simulink library "csu_prb_orbit_perturbations_model_lib"  (R2014b)
settings: Solver=ode45  SolverMode=SingleTasking  StartTime=0.0  StopTime=10.0  RelTol=1e-3
values from neighbouring files (symbols this model uses):
  grv_mu_moon = gbl_param.moon_gravity_mu    [csu_grs_gravity_r_squared_init.m]
  ini_epoch_seconds = gbl_param.epoch_seconds    [csu_ini_initial_conditions_init.m]
undefined symbols (not defined in the file or in its folder): pos_s2m_mcmf, prb_gg_torque_on, prb_srp_force_on, r_moon, r_sun, spice_time_step_size, srp_K
libraries: util_common_lib x11, util_info_lib x7, util_quat_lib x4, csu_prb_orbit_perturbations_model_lib x2, csu_srp_solar_radiation_model_lib x1
settings Model: ExtModeAutoUpdateStatusClock=off  Creator=daniloviazzo  LastModifiedBy=mstewart

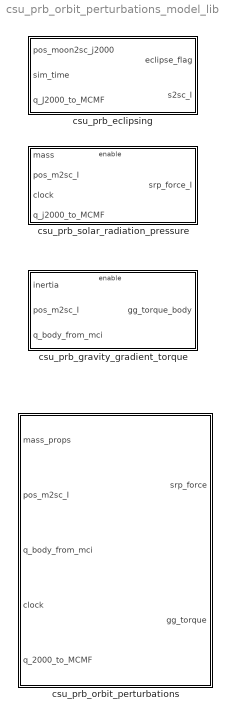
== system csu_prb_orbit_perturbations_model_lib ==
  csu_prb_eclipsing : Subsystem
  csu_prb_gravity_gradient_torque : Subsystem
  csu_prb_orbit_perturbations : Subsystem
  csu_prb_solar_radiation_pressure : Subsystem

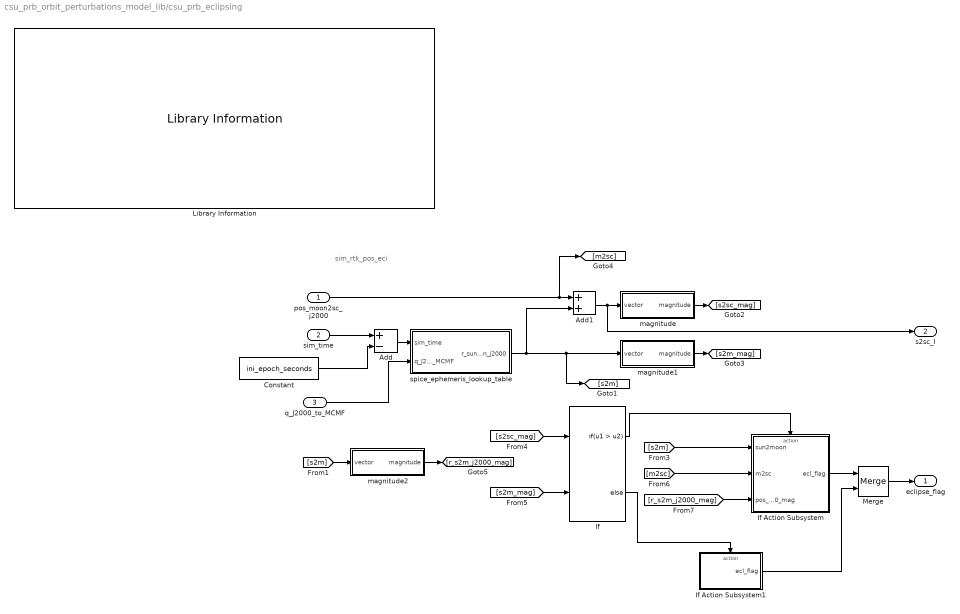
== system csu_prb_orbit_perturbations_model_lib/csu_prb_eclipsing ==
  note: sim_rtk_pos_eci
  pos_moon2sc_j2000 : Inport
  sim_time : Inport  Port=2
  q_J2000_to_MCMF : Inport  Port=3
  Add : Sum  Inputs=+-
  Add1 : Sum
  Constant : Constant  Value=ini_epoch_seconds
  If : If  NumInputs=2  IfExpression=u1 > u2
  If Action Subsystem : Subsystem  TreatAsAtomicUnit=on
  If Action Subsystem1 : Subsystem  TreatAsAtomicUnit=on
  Library Information : util_info_lib/Library Information  owner='NONE'
  Merge : Merge
  magnitude : Subsystem
  magnitude1 : Subsystem
  magnitude2 : Subsystem
  spice_ephemeris_lookup_table : Subsystem
  eclipse_flag : Outport
  s2sc_I : Outport  Port=2
  wires:
  [m2sc] -> If Action Subsystem/2(m2sc)
  [s2m_mag] -> If/2
  [s2sc_mag] -> If/1
  magnitude1/1(magnitude) -> [s2m_mag]
  magnitude/1(magnitude) -> [s2sc_mag]
  [s2m] -> If Action Subsystem/1(sun2moon)
  spice_ephemeris_lookup_table/1(r_sun2moon_j2000) -> magnitude1/1(vector), [s2m], Add1/2
  Add1/1 -> s2sc_I/1, magnitude/1(vector)
  Merge/1 -> eclipse_flag/1
  If Action Subsystem/1(ecl_flag) -> Merge/1
  If Action Subsystem1/1(ecl_flag) -> Merge/2
  If/2 -> If Action Subsystem1/Action
  If/1 -> If Action Subsystem/Action
  pos_moon2sc_j2000/1 -> [m2sc], Add1/1
  sim_time/1 -> Add/1
  Constant/1 -> Add/2
  Add/1 -> spice_ephemeris_lookup_table/1(sim_time)
  [r_s2m_j2000_mag] -> If Action Subsystem/3(pos_s2m_j2000_mag)
  q_J2000_to_MCMF/1 -> spice_ephemeris_lookup_table/2(q_J2000_to_MCMF)
  magnitude2/1(magnitude) -> [r_s2m_j2000_mag]
  [s2m] -> magnitude2/1(vector)

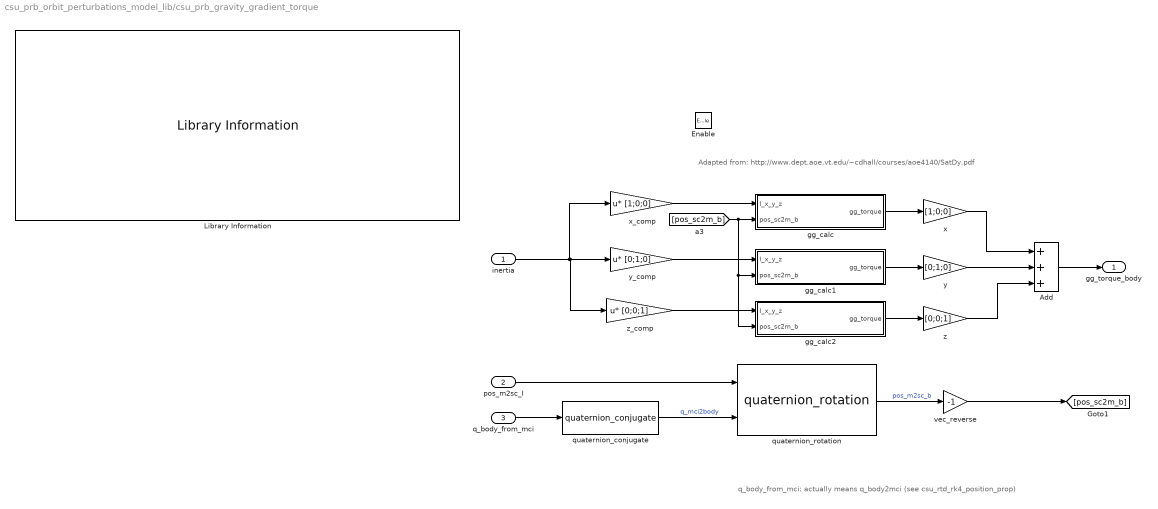
== system csu_prb_orbit_perturbations_model_lib/csu_prb_gravity_gradient_torque ==
  note: Adapted from: http://www.dept.aoe.vt.edu/~cdhall/courses/aoe4140/SatDy.pdf
  note: q_body_from_mci: actually means q_body2mci (see csu_rtd_rk4_position_prop)
  inertia : Inport
  pos_m2sc_I : Inport  Port=2
  q_body_from_mci : Inport  Port=3
  Enable : EnablePort
  Add : Sum  Inputs=+++
  Library Information : util_info_lib/Library Information  owner='NONE'
  gg_calc : Subsystem
  gg_calc1 : Subsystem
  gg_calc2 : Subsystem
  quaternion_conjugate : util_quat_lib/quaternion_conjugate  SystemSampleTime=-1
  quaternion_rotation : util_quat_lib/quaternion_rotation  SystemSampleTime=-1
  vec_reverse : Gain  Gain=-1
  x : Gain  Gain=[1;0;0]
  x_comp : Gain  Gain=[1;0;0]  Multiplication=Matrix(u*K)
  y : Gain  Gain=[0;1;0]
  y_comp : Gain  Gain=[0;1;0]  Multiplication=Matrix(u*K)
  z : Gain  Gain=[0;0;1]
  z_comp : Gain  Gain=[0;0;1]  Multiplication=Matrix(u*K)
  gg_torque_body : Outport
  wires:
  gg_calc2/1(gg_torque) -> z/1
  gg_calc1/1(gg_torque) -> y/1
  gg_calc/1(gg_torque) -> x/1
  [pos_sc2m_b] -> gg_calc/2(pos_sc2m_b), gg_calc1/2(pos_sc2m_b), gg_calc2/2(pos_sc2m_b)
  z_comp/1 -> gg_calc2/1(I_x_y_z)
  y_comp/1 -> gg_calc1/1(I_x_y_z)
  x_comp/1 -> gg_calc/1(I_x_y_z)
  Add/1 -> gg_torque_body/1
  inertia/1 -> y_comp/1, z_comp/1, x_comp/1
  vec_reverse/1 -> [pos_sc2m_b]
  quaternion_rotation/1 -> vec_reverse/1  "pos_m2sc_b"
  quaternion_conjugate/1 -> quaternion_rotation/2  "q_mci2body"
  q_body_from_mci/1 -> quaternion_conjugate/1
  pos_m2sc_I/1 -> quaternion_rotation/1
  x/1 -> Add/1
  y/1 -> Add/2
  z/1 -> Add/3

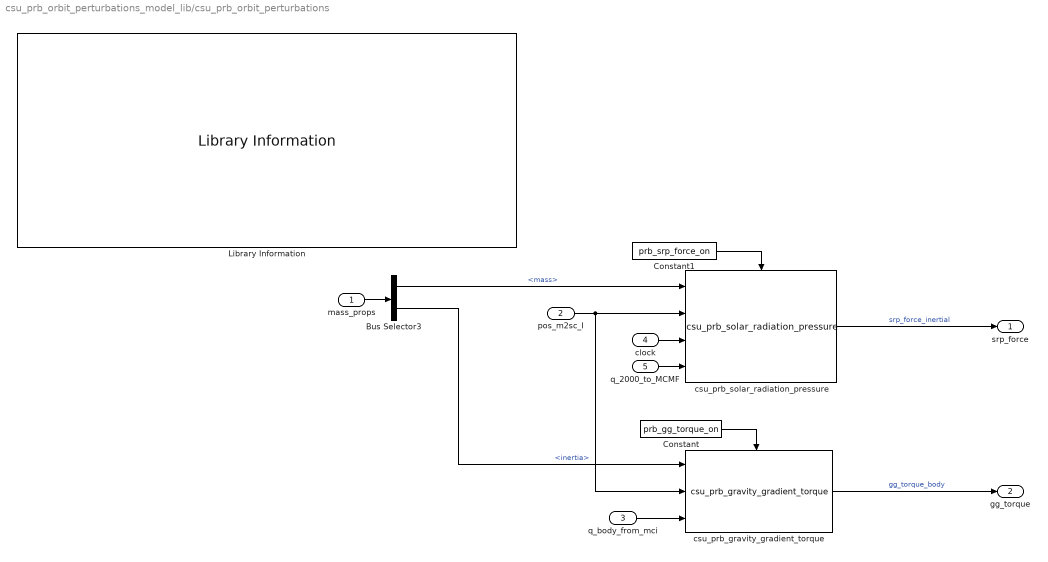
== system csu_prb_orbit_perturbations_model_lib/csu_prb_orbit_perturbations ==
  mass_props : Inport
  pos_m2sc_I : Inport  Port=2
  q_body_from_mci : Inport  Port=3
  clock : Inport  Port=4
  q_2000_to_MCMF : Inport  Port=5
  Bus Selector3 : BusSelector  OutputSignals=mass,inertia
  Constant : Constant  Value=prb_gg_torque_on
  Constant1 : Constant  Value=prb_srp_force_on
  Library Information : util_info_lib/Library Information  owner='NONE'
  csu_prb_gravity_gradient_torque : csu_prb_orbit_perturbations_model_lib/csu_prb_gravity_gradient_torque
  csu_prb_solar_radiation_pressure : csu_prb_orbit_perturbations_model_lib/csu_prb_solar_radiation_pressure
  srp_force : Outport
  gg_torque : Outport  Port=2
  wires:
  Bus Selector3/1 -> csu_prb_solar_radiation_pressure/1  "<mass>"
  mass_props/1 -> Bus Selector3/1
  q_2000_to_MCMF/1 -> csu_prb_solar_radiation_pressure/4
  clock/1 -> csu_prb_solar_radiation_pressure/3
  pos_m2sc_I/1 -> csu_prb_solar_radiation_pressure/2, csu_prb_gravity_gradient_torque/2
  q_body_from_mci/1 -> csu_prb_gravity_gradient_torque/3
  Constant/1 -> csu_prb_gravity_gradient_torque/Enable
  Constant1/1 -> csu_prb_solar_radiation_pressure/Enable
  Bus Selector3/2 -> csu_prb_gravity_gradient_torque/1  "<inertia>"
  csu_prb_solar_radiation_pressure/1 -> srp_force/1  "srp_force_inertial"
  csu_prb_gravity_gradient_torque/1 -> gg_torque/1  "gg_torque_body"

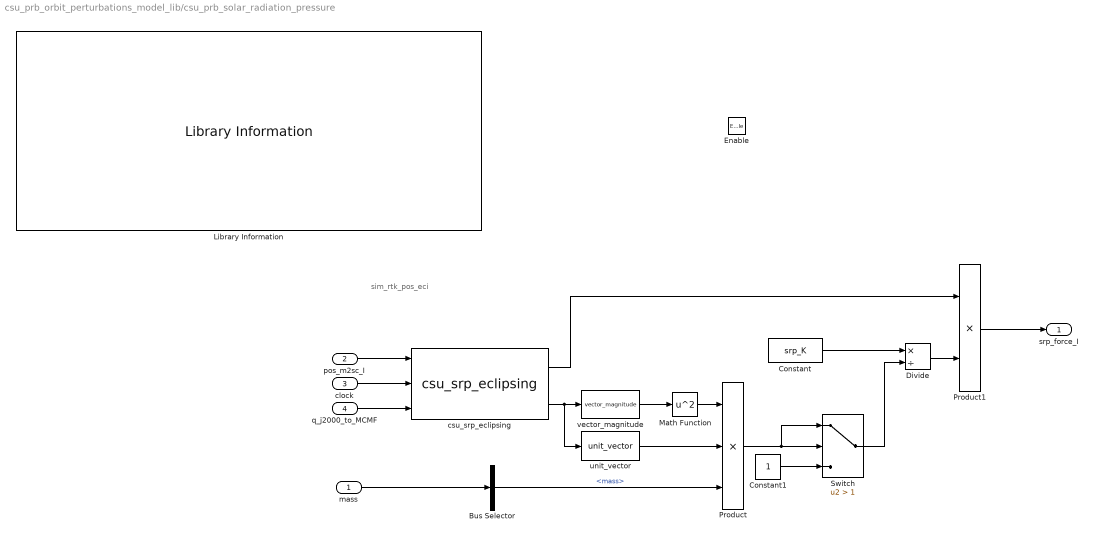
== system csu_prb_orbit_perturbations_model_lib/csu_prb_solar_radiation_pressure ==
  note: sim_rtk_pos_eci
  mass : Inport
  pos_m2sc_I : Inport  Port=2
  clock : Inport  Port=3
  q_j2000_to_MCMF : Inport  Port=4
  Enable : EnablePort
  Bus Selector : BusSelector  OutputSignals=mass
  Constant : Constant  Value=srp_K
  Constant1 : Constant
  Divide : Product  Inputs=*/
  Library Information : util_info_lib/Library Information  owner='NONE'
  Math Function : Math  Operator=square  SaturateOnIntegerOverflow=on
  Product : Product  Inputs=3
  Product1 : Product
  Switch : Switch  Criteria=u2 > Threshold  Threshold=1
  csu_srp_eclipsing : csu_srp_solar_radiation_model_lib/csu_srp_eclipsing
  unit_vector : util_common_lib/unit_vector  SystemSampleTime=-1
  vector_magnitude : util_common_lib/vector_magnitude  SystemSampleTime=-1
  srp_force_I : Outport
  wires:
  Constant/1 -> Divide/1
  pos_m2sc_I/1 -> csu_srp_eclipsing/1
  clock/1 -> csu_srp_eclipsing/2
  q_j2000_to_MCMF/1 -> csu_srp_eclipsing/3
  csu_srp_eclipsing/1 -> Product1/1
  csu_srp_eclipsing/2 -> vector_magnitude/1, unit_vector/1
  vector_magnitude/1 -> Math Function/1
  mass/1 -> Bus Selector/1
  Product/1 -> Switch/2, Switch/1
  Switch/1 -> Divide/2
  Constant1/1 -> Switch/3
  Divide/1 -> Product1/2
  Product1/1 -> srp_force_I/1
  Math Function/1 -> Product/1
  unit_vector/1 -> Product/2
  Bus Selector/1 -> Product/3  "<mass>"

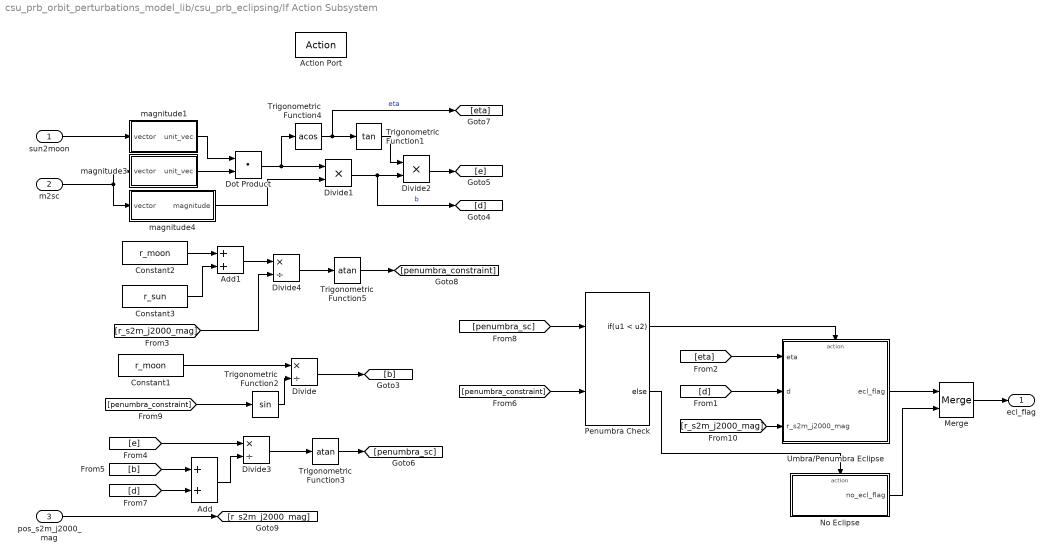
== system csu_prb_orbit_perturbations_model_lib/csu_prb_eclipsing/If Action Subsystem ==
  sun2moon : Inport
  m2sc : Inport  Port=2
  pos_s2m_j2000_mag : Inport  Port=3
  Action Port : ActionPort
  Add : Sum
  Add1 : Sum
  Constant1 : Constant  Value=r_moon
  Constant2 : Constant  Value=r_moon
  Constant3 : Constant  Value=r_sun
  Divide : Product  Inputs=*/
  Divide1 : Product  Inputs=**
  Divide2 : Product  Inputs=**
  Divide3 : Product  Inputs=*/
  Divide4 : Product  Inputs=*/
  Dot Product : DotProduct  InputSameDT=on  OutDataTypeStr=Inherit: Inherit via internal rule
  Merge : Merge
  No Eclipse : Subsystem  TreatAsAtomicUnit=on
  Penumbra Check : If  NumInputs=2  IfExpression=u1 < u2
  Trigonometric Function1 : Trigonometry  Operator=tan
  Trigonometric Function2 : Trigonometry
  Trigonometric Function3 : Trigonometry  Operator=atan
  Trigonometric Function4 : Trigonometry  Operator=acos
  Trigonometric Function5 : Trigonometry  Operator=atan
  Umbra/Penumbra Eclipse : Subsystem  TreatAsAtomicUnit=on
  magnitude1 : Subsystem
  magnitude3 : Subsystem
  magnitude4 : Subsystem
  ecl_flag : Outport
  wires:
  [penumbra_sc] -> Penumbra Check/1
  Umbra/Penumbra Eclipse/1(ecl_flag) -> Merge/1
  Merge/1 -> ecl_flag/1
  No Eclipse/1(no_ecl_flag) -> Merge/2
  Penumbra Check/2 -> No Eclipse/Action
  Penumbra Check/1 -> Umbra/Penumbra Eclipse/Action
  [d] -> Umbra/Penumbra Eclipse/2(d)
  m2sc/1 -> magnitude3/1(vector), magnitude4/1(vector)
  magnitude4/1(magnitude) -> Divide1/2
  magnitude1/1(unit_vec) -> Dot Product/1
  magnitude3/1(unit_vec) -> Dot Product/2
  sun2moon/1 -> magnitude1/1(vector)
  Dot Product/1 -> Trigonometric Function4/1, Divide1/1
  Divide2/1 -> [e]
  Trigonometric Function1/1 -> Divide2/1
  [penumbra_constraint] -> Trigonometric Function2/1
  Constant1/1 -> Divide/1
  Trigonometric Function2/1 -> Divide/2
  Divide/1 -> [b]
  [e] -> Divide3/1
  Divide1/1 -> [d], Divide2/2  "b"
  [b] -> Add/1
  [d] -> Add/2
  Add/1 -> Divide3/2
  Divide3/1 -> Trigonometric Function3/1
  Trigonometric Function3/1 -> [penumbra_sc]
  Trigonometric Function4/1 -> [eta], Trigonometric Function1/1  "eta"
  [eta] -> Umbra/Penumbra Eclipse/1(eta)
  pos_s2m_j2000_mag/1 -> [r_s2m_j2000_mag]
  [penumbra_constraint] -> Penumbra Check/2
  [r_s2m_j2000_mag] -> Umbra/Penumbra Eclipse/3("r_s2m_j2000_mag ")
  Constant2/1 -> Add1/1
  Constant3/1 -> Add1/2
  Add1/1 -> Divide4/1
  Divide4/1 -> Trigonometric Function5/1
  Trigonometric Function5/1 -> [penumbra_constraint]
  [r_s2m_j2000_mag] -> Divide4/2

== system csu_prb_orbit_perturbations_model_lib/csu_prb_eclipsing/If Action Subsystem1 ==
  Action Port : ActionPort
  Constant : Constant  Value=0
  ecl_flag : Outport
  wires:
  Constant/1 -> ecl_flag/1

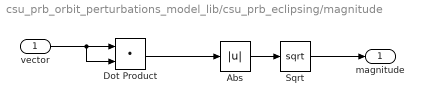
== system csu_prb_orbit_perturbations_model_lib/csu_prb_eclipsing/magnitude ==
  vector : Inport
  Abs : Abs
  Dot Product : DotProduct  InputSameDT=on  OutDataTypeStr=Inherit: Inherit via internal rule
  Sqrt : Sqrt  SaturateOnIntegerOverflow=on
  magnitude : Outport
  wires:
  Abs/1 -> Sqrt/1
  Sqrt/1 -> magnitude/1
  Dot Product/1 -> Abs/1
  vector/1 -> Dot Product/1, Dot Product/2

== system csu_prb_orbit_perturbations_model_lib/csu_prb_eclipsing/magnitude1 ==
  vector : Inport
  Abs : Abs
  Dot Product : DotProduct  InputSameDT=on  OutDataTypeStr=Inherit: Inherit via internal rule
  Sqrt : Sqrt  SaturateOnIntegerOverflow=on
  magnitude : Outport
  wires:
  vector/1 -> Dot Product/2, Dot Product/1
  Dot Product/1 -> Abs/1
  Sqrt/1 -> magnitude/1
  Abs/1 -> Sqrt/1

== system csu_prb_orbit_perturbations_model_lib/csu_prb_eclipsing/magnitude2 ==
  vector : Inport
  Abs : Abs
  Dot Product : DotProduct  InputSameDT=on  OutDataTypeStr=Inherit: Inherit via internal rule
  Sqrt : Sqrt  SaturateOnIntegerOverflow=on
  magnitude : Outport
  wires:
  vector/1 -> Dot Product/2, Dot Product/1
  Dot Product/1 -> Abs/1
  Sqrt/1 -> magnitude/1
  Abs/1 -> Sqrt/1

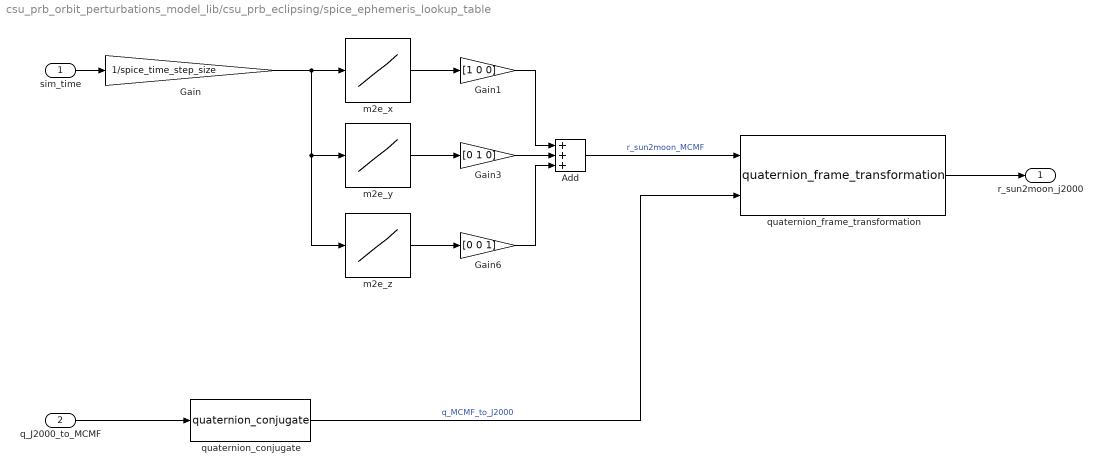
== system csu_prb_orbit_perturbations_model_lib/csu_prb_eclipsing/spice_ephemeris_lookup_table ==
  sim_time : Inport
  q_J2000_to_MCMF : Inport  Port=2
  Add : Sum  Inputs=+++
  Gain : Gain  Gain=1/spice_time_step_size
  Gain1 : Gain  Gain=[1 0 0]
  Gain3 : Gain  Gain=[0 1 0]
  Gain6 : Gain  Gain=[0 0 1]
  m2e_x : Lookup_n-D  NumberOfTableDimensions=1  BreakpointsForDimension1=[1:length(pos_s2m_mcmf)]  Table=pos_s2m_mcmf(:,1)  RndMeth=Simplest  InputSameDT=on
  m2e_y : Lookup_n-D  NumberOfTableDimensions=1  BreakpointsForDimension1=[1:length(pos_s2m_mcmf)]  Table=pos_s2m_mcmf(:,2)  RndMeth=Simplest  InputSameDT=on
  m2e_z : Lookup_n-D  NumberOfTableDimensions=1  BreakpointsForDimension1=[1:length(pos_s2m_mcmf)]  Table=pos_s2m_mcmf(:,3)  RndMeth=Simplest  InputSameDT=on
  quaternion_conjugate : util_quat_lib/quaternion_conjugate  SystemSampleTime=-1
  quaternion_frame_transformation : util_quat_lib/quaternion_frame_transformation  SystemSampleTime=-1
  r_sun2moon_j2000 : Outport
  wires:
  sim_time/1 -> Gain/1
  m2e_x/1 -> Gain1/1
  Gain/1 -> m2e_z/1, m2e_y/1, m2e_x/1
  m2e_y/1 -> Gain3/1
  m2e_z/1 -> Gain6/1
  Gain3/1 -> Add/2
  Gain1/1 -> Add/1
  Gain6/1 -> Add/3
  q_J2000_to_MCMF/1 -> quaternion_conjugate/1
  quaternion_frame_transformation/1 -> r_sun2moon_j2000/1
  quaternion_conjugate/1 -> quaternion_frame_transformation/2  "q_MCMF_to_J2000"
  Add/1 -> quaternion_frame_transformation/1  "r_sun2moon_MCMF"

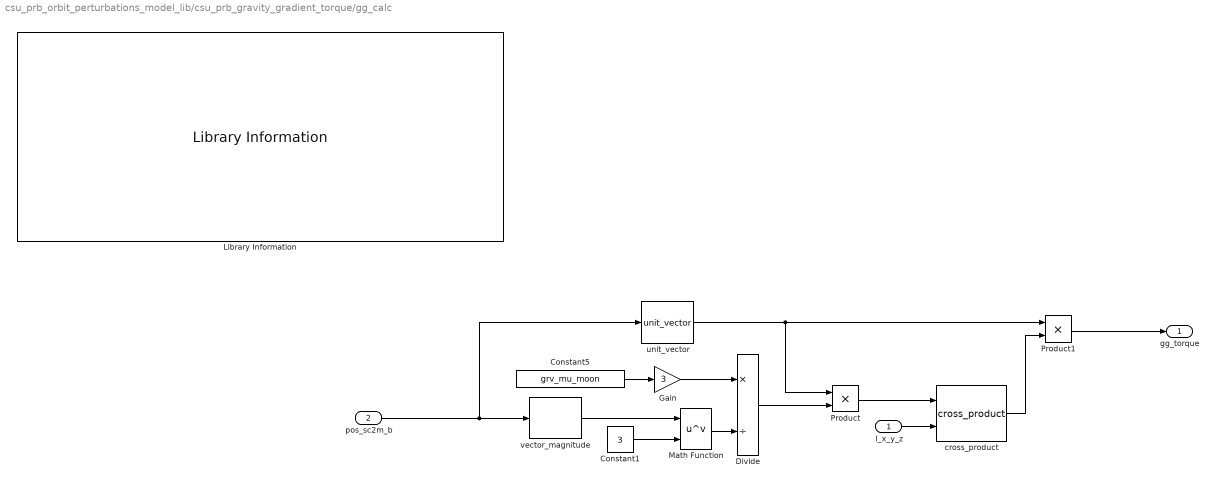
== system csu_prb_orbit_perturbations_model_lib/csu_prb_gravity_gradient_torque/gg_calc ==
  I_x_y_z : Inport
  pos_sc2m_b : Inport  Port=2
  Constant1 : Constant  Value=3
  Constant5 : Constant  Value=grv_mu_moon
  Divide : Product  Inputs=*/
  Gain : Gain  Gain=3
  Library Information : util_info_lib/Library Information  owner='NONE'
  Math Function : Math  Operator=pow  SaturateOnIntegerOverflow=on
  Product : Product
  Product1 : Product
  cross_product : util_common_lib/cross_product  SystemSampleTime=-1
  unit_vector : util_common_lib/unit_vector  SystemSampleTime=-1
  vector_magnitude : util_common_lib/vector_magnitude  SystemSampleTime=-1
  gg_torque : Outport
  wires:
  Product1/1 -> gg_torque/1
  pos_sc2m_b/1 -> vector_magnitude/1, unit_vector/1
  unit_vector/1 -> Product/1, Product1/1
  Math Function/1 -> Divide/2
  Gain/1 -> Divide/1
  Constant5/1 -> Gain/1
  Constant1/1 -> Math Function/2
  vector_magnitude/1 -> Math Function/1
  I_x_y_z/1 -> cross_product/2
  cross_product/1 -> Product1/2
  Divide/1 -> Product/2
  Product/1 -> cross_product/1

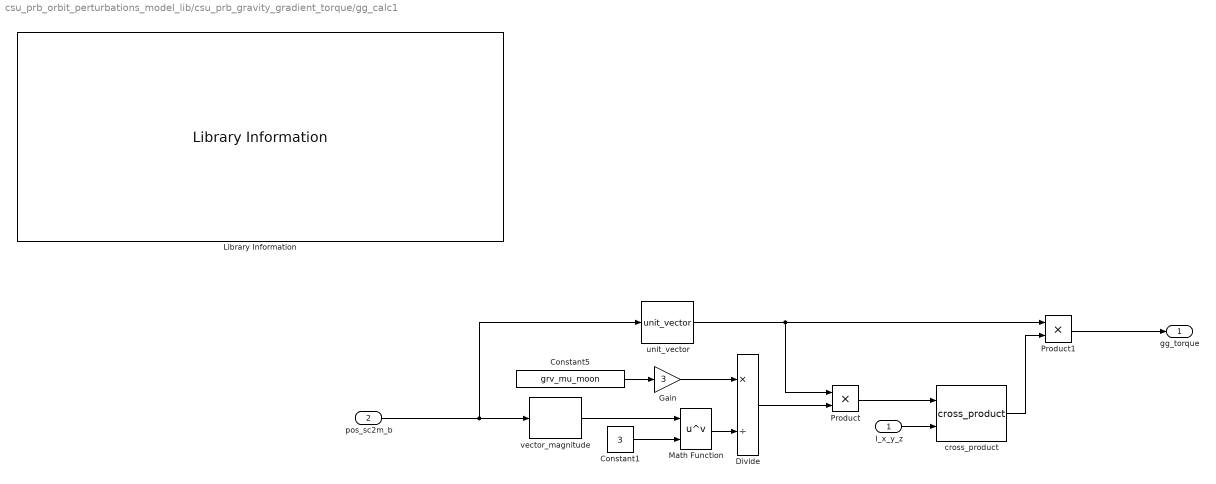
== system csu_prb_orbit_perturbations_model_lib/csu_prb_gravity_gradient_torque/gg_calc1 ==
  I_x_y_z : Inport
  pos_sc2m_b : Inport  Port=2
  Constant1 : Constant  Value=3
  Constant5 : Constant  Value=grv_mu_moon
  Divide : Product  Inputs=*/
  Gain : Gain  Gain=3
  Library Information : util_info_lib/Library Information  owner='NONE'
  Math Function : Math  Operator=pow  SaturateOnIntegerOverflow=on
  Product : Product
  Product1 : Product
  cross_product : util_common_lib/cross_product  SystemSampleTime=-1
  unit_vector : util_common_lib/unit_vector  SystemSampleTime=-1
  vector_magnitude : util_common_lib/vector_magnitude  SystemSampleTime=-1
  gg_torque : Outport
  wires:
  Product1/1 -> gg_torque/1
  pos_sc2m_b/1 -> vector_magnitude/1, unit_vector/1
  unit_vector/1 -> Product/1, Product1/1
  Math Function/1 -> Divide/2
  Gain/1 -> Divide/1
  Constant5/1 -> Gain/1
  Constant1/1 -> Math Function/2
  vector_magnitude/1 -> Math Function/1
  I_x_y_z/1 -> cross_product/2
  cross_product/1 -> Product1/2
  Divide/1 -> Product/2
  Product/1 -> cross_product/1

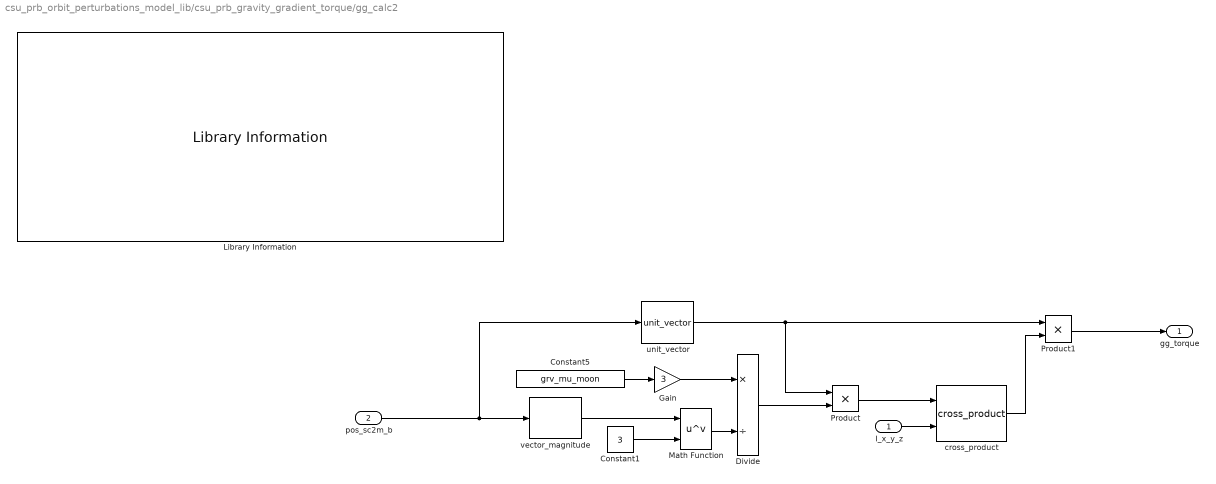
== system csu_prb_orbit_perturbations_model_lib/csu_prb_gravity_gradient_torque/gg_calc2 ==
  I_x_y_z : Inport
  pos_sc2m_b : Inport  Port=2
  Constant1 : Constant  Value=3
  Constant5 : Constant  Value=grv_mu_moon
  Divide : Product  Inputs=*/
  Gain : Gain  Gain=3
  Library Information : util_info_lib/Library Information  owner='NONE'
  Math Function : Math  Operator=pow  SaturateOnIntegerOverflow=on
  Product : Product
  Product1 : Product
  cross_product : util_common_lib/cross_product  SystemSampleTime=-1
  unit_vector : util_common_lib/unit_vector  SystemSampleTime=-1
  vector_magnitude : util_common_lib/vector_magnitude  SystemSampleTime=-1
  gg_torque : Outport
  wires:
  Product1/1 -> gg_torque/1
  pos_sc2m_b/1 -> vector_magnitude/1, unit_vector/1
  unit_vector/1 -> Product/1, Product1/1
  Math Function/1 -> Divide/2
  Gain/1 -> Divide/1
  Constant5/1 -> Gain/1
  Constant1/1 -> Math Function/2
  vector_magnitude/1 -> Math Function/1
  I_x_y_z/1 -> cross_product/2
  cross_product/1 -> Product1/2
  Divide/1 -> Product/2
  Product/1 -> cross_product/1

== system csu_prb_orbit_perturbations_model_lib/csu_prb_eclipsing/If Action Subsystem/No Eclipse ==
  Action Port : ActionPort
  Constant : Constant  Value=0
  no_ecl_flag : Outport
  wires:
  Constant/1 -> no_ecl_flag/1

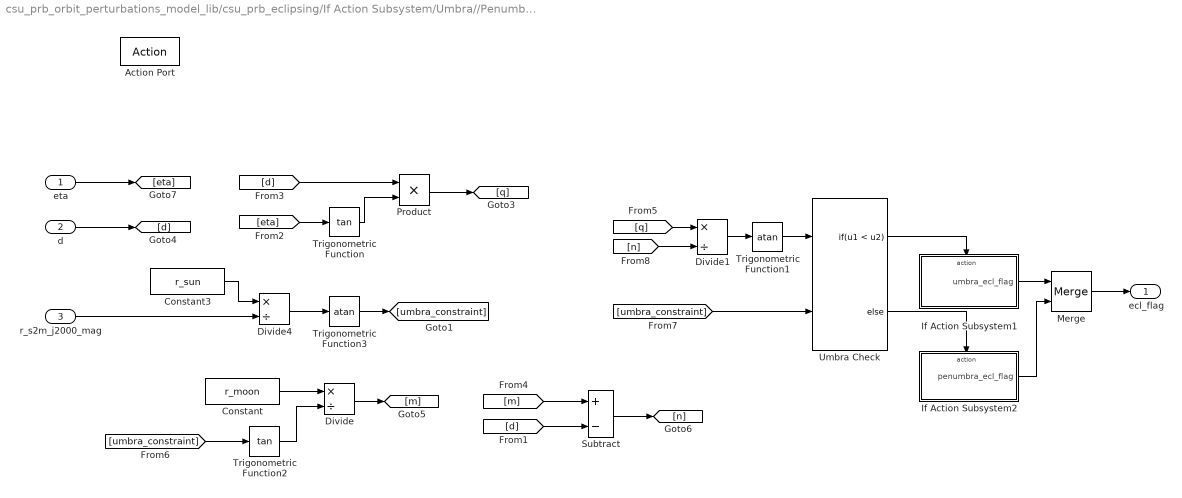
== system csu_prb_orbit_perturbations_model_lib/csu_prb_eclipsing/If Action Subsystem/Umbra//Penumbra Eclipse ==
  eta : Inport
  d : Inport  Port=2
  "r_s2m_j2000_mag " : Inport  Port=3
  Action Port : ActionPort
  Constant : Constant  Value=r_moon
  Constant3 : Constant  Value=r_sun
  Divide : Product  Inputs=*/
  Divide1 : Product  Inputs=*/
  Divide4 : Product  Inputs=*/
  If Action Subsystem1 : Subsystem  TreatAsAtomicUnit=on
  If Action Subsystem2 : Subsystem  TreatAsAtomicUnit=on
  Merge : Merge
  Product : Product
  Subtract : Sum  Inputs=+-
  Trigonometric Function : Trigonometry  Operator=tan
  Trigonometric Function1 : Trigonometry  Operator=atan
  Trigonometric Function2 : Trigonometry  Operator=tan
  Trigonometric Function3 : Trigonometry  Operator=atan
  Umbra Check : If  NumInputs=2  IfExpression=u1 < u2
  ecl_flag : Outport
  wires:
  Merge/1 -> ecl_flag/1
  If Action Subsystem2/1(penumbra_ecl_flag) -> Merge/2
  Umbra Check/2 -> If Action Subsystem2/Action
  If Action Subsystem1/1(umbra_ecl_flag) -> Merge/1
  Umbra Check/1 -> If Action Subsystem1/Action
  eta/1 -> [eta]
  d/1 -> [d]
  Constant/1 -> Divide/1
  Divide/1 -> [m]
  [m] -> Subtract/1
  [d] -> Subtract/2
  [eta] -> Trigonometric Function/1
  [d] -> Product/1
  Trigonometric Function/1 -> Product/2
  Product/1 -> [q]
  Subtract/1 -> [n]
  [q] -> Divide1/1
  [n] -> Divide1/2
  Divide1/1 -> Trigonometric Function1/1
  Trigonometric Function1/1 -> Umbra Check/1
  [umbra_constraint] -> Trigonometric Function2/1
  [umbra_constraint] -> Umbra Check/2
  Trigonometric Function2/1 -> Divide/2
  Constant3/1 -> Divide4/1
  "r_s2m_j2000_mag "/1 -> Divide4/2
  Divide4/1 -> Trigonometric Function3/1
  Trigonometric Function3/1 -> [umbra_constraint]

== system csu_prb_orbit_perturbations_model_lib/csu_prb_eclipsing/If Action Subsystem/magnitude1 ==
  vector : Inport
  Divide : Product  Inputs=*/
  magnitude1 : Subsystem
  unit_vec : Outport
  wires:
  Divide/1 -> unit_vec/1
  magnitude1/1(magnitude) -> Divide/2
  vector/1 -> magnitude1/1(vector), Divide/1

== system csu_prb_orbit_perturbations_model_lib/csu_prb_eclipsing/If Action Subsystem/magnitude3 ==
  vector : Inport
  Divide : Product  Inputs=*/
  magnitude1 : Subsystem
  unit_vec : Outport
  wires:
  vector/1 -> Divide/1, magnitude1/1(vector)
  magnitude1/1(magnitude) -> Divide/2
  Divide/1 -> unit_vec/1

== system csu_prb_orbit_perturbations_model_lib/csu_prb_eclipsing/If Action Subsystem/magnitude4 ==
  vector : Inport
  Abs : Abs
  Dot Product : DotProduct  InputSameDT=on  OutDataTypeStr=Inherit: Inherit via internal rule
  Sqrt : Sqrt  SaturateOnIntegerOverflow=on
  magnitude : Outport
  wires:
  Abs/1 -> Sqrt/1
  Sqrt/1 -> magnitude/1
  Dot Product/1 -> Abs/1
  vector/1 -> Dot Product/1, Dot Product/2

== system csu_prb_orbit_perturbations_model_lib/csu_prb_eclipsing/If Action Subsystem/Umbra//Penumbra Eclipse/If Action Subsystem1 ==
  note: (nested if statement)
  Action Port : ActionPort
  Constant : Constant
  umbra_ecl_flag : Outport
  wires:
  Constant/1 -> umbra_ecl_flag/1

== system csu_prb_orbit_perturbations_model_lib/csu_prb_eclipsing/If Action Subsystem/Umbra//Penumbra Eclipse/If Action Subsystem2 ==
  Action Port : ActionPort
  Constant : Constant  Value=0.5
  penumbra_ecl_flag : Outport
  wires:
  Constant/1 -> penumbra_ecl_flag/1

== system csu_prb_orbit_perturbations_model_lib/csu_prb_eclipsing/If Action Subsystem/magnitude1/magnitude1 ==
  vector : Inport
  Abs : Abs
  Dot Product : DotProduct  InputSameDT=on  OutDataTypeStr=Inherit: Inherit via internal rule
  Sqrt : Sqrt  SaturateOnIntegerOverflow=on
  magnitude : Outport
  wires:
  vector/1 -> Dot Product/2, Dot Product/1
  Dot Product/1 -> Abs/1
  Sqrt/1 -> magnitude/1
  Abs/1 -> Sqrt/1

== system csu_prb_orbit_perturbations_model_lib/csu_prb_eclipsing/If Action Subsystem/magnitude3/magnitude1 ==
  vector : Inport
  Abs : Abs
  Dot Product : DotProduct  InputSameDT=on  OutDataTypeStr=Inherit: Inherit via internal rule
  Sqrt : Sqrt  SaturateOnIntegerOverflow=on
  magnitude : Outport
  wires:
  Abs/1 -> Sqrt/1
  Sqrt/1 -> magnitude/1
  Dot Product/1 -> Abs/1
  vector/1 -> Dot Product/1, Dot Product/2
